simulink model "Fly_calculatedLm"  (R2017b)
settings: Solver=VariableStepAuto  StartTime=0.0  StopTime=1  MaxStep=1e-4  RelTol=1e-3
libraries: powerlib x17, powerlib_meascontrol x1
settings Model: Creator=yusuf  LastModifiedBy=SiF
settings CodeAppCC: StateflowObjectComments=on

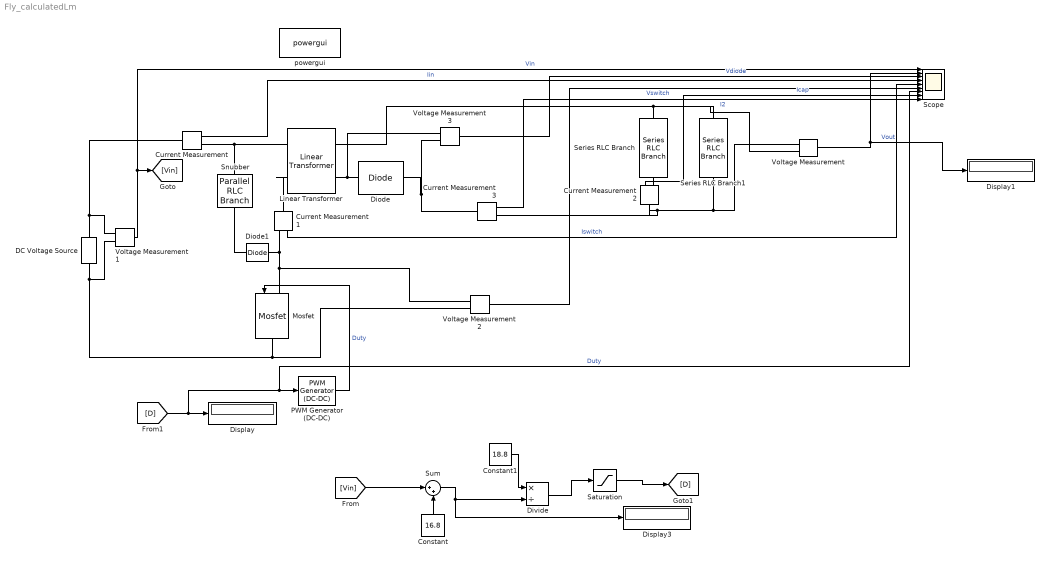
== system Fly_calculatedLm ==
  Constant : Constant  Value=16.8
  Constant1 : Constant  Value=18.8
  Current Measurement{,1..3} (4 alike) : powerlib/Measurements/Current Measurement  PhasorSimulation=off  OutputType=Complex  PSBequivalent=0
  DC Voltage Source : powerlib/Electrical Sources/DC Voltage Source  Amplitude=48  Measurements=None
  Diode : powerlib/Power Electronics/Diode  Ron=0.001  Lon=0  Vf=0.8  IC=0  UseSnubber=0  Rs=500  Cs=250e-9  Measurements=off
  Diode1 : powerlib/Power Electronics/Diode  Ron=0.001  Lon=0  Vf=0.8  IC=0  UseSnubber=0  Rs=500  Cs=250e-9  Measurements=off
  Display : Display
  Display1 : Display
  Display3 : Display
  Divide : Product  Inputs=*/
  Linear Transformer : powerlib/Elements/Linear Transformer  UNITS=SI  NominalPower=[100 32e3 ]  winding1=[60 0 12e-6]  winding2=[20 0 0]  ThreeWindings=off  winding3=[3.15e+05 0.7938 0.0001316]  RmLm=[1080.5 400e-6]  Measurements=Magnetization current  DataType=on
  Mosfet : powerlib/Power Electronics/Mosfet  Ron=0.1  Lon=0  Rd=0.01  Vfd=0  IC=0  Rs=1e5  Cs=inf  Measurements=off
  PWM Generator (DC-DC) : powerlib_meascontrol/Pulse & Signal Generators/PWM Generator (DC-DC)  Fsw=32000  Ts=0
  Saturation : Saturate  UpperLimit=0.85  LowerLimit=0
  Scope : Scope  NumInputPorts=9
  Series RLC Branch : powerlib/Elements/Series RLC Branch  LConnTagsString=__new0  RConnTagsString=__new0  BranchType=C  Resistance=1  Inductance=1e-3  SetiL0=off  InitialCurrent=0  Capacitance=1e-3  Setx0=off  InitialVoltage=0  Measurements=None
  Series RLC Branch1 : powerlib/Elements/Series RLC Branch  LConnTagsString=__new0  RConnTagsString=__new0  BranchType=R  Resistance=5/6  Inductance=1e-3  SetiL0=off  InitialCurrent=0  Capacitance=1e-6  Setx0=off  InitialVoltage=0  Measurements=None
  Snubber : powerlib/Elements/Parallel RLC Branch  LConnTagsString=a  RConnTagsString=__new0  BranchType=RC  Resistance=10e3  Inductance=1e-3  SetiL0=off  InitialCurrent=0  Capacitance=47e-9  Setx0=off  InitialVoltage=0  Measurements=None
  Sum : Sum  Inputs=|++
  Voltage Measurement{,1..3} (4 alike) : powerlib/Measurements/Voltage Measurement  PhasorSimulation=off  OutputType=Complex  PSBequivalent=0
  powergui : powerlib/powergui  Priority=1  SimulationMode=Continuous  SampleTime=50e-6  frequency=60  Iterations=50  frequencyindice=0  Pbase=100e6  ErrMax=1e-4  UnitsV=kV  UnitsW=MW  buscounter=0  FunctionMessages=off  echomessages=off  EnableUseOfTLC=off  CurrentSourceSwitches=off  DisableSnubberDevices=off  DisableRonSwitches=off  DisableVfSwitches=off  DisplayEquations=off  SolverType=Tustin/Backward Euler (TBE)  Interpol=off  ExternalGateDelay=off  methode=off  Ts=100  x0status=blocks  SPID=on  SwTol=0  HookPort=off  RestoreLinks=warning  ResistiveCurrentMeasurement=off  Frange=[0:2:500]  Ylog=off  Xlog=on  ShowGrid=off  save=off  variable=ZData  structure=0  ZoomFFT=off  StartTime=0.0  cycles=1  DisplayStyle=1  fundamental=60  FreqAxis=off  MaxFrequency=1000  frequencyindicesteady=1  RmsSteady=1  display=off
  wires:
  [D] -> Display/1, Scope/7, PWM Generator (DC-DC)/1  "Duty"
  PWM Generator (DC-DC)/1 -> Mosfet/1  "Duty"
  Voltage Measurement/1 -> Display1/1, Scope/2  "Vout"
  Current Measurement/1 -> Scope/4  "Iin"
  Voltage Measurement1/1 -> [Vin], Scope/1  "Vin"
  Current Measurement1/1 -> Scope/5  "Iswitch"
  Voltage Measurement2/1 -> Scope/6  "Vswitch"
  Current Measurement2/1 -> Scope/8  "Icap"
  [Vin] -> Sum/1
  Constant/1 -> Sum/2
  Sum/1 -> Divide/2, Display3/1
  Saturation/1 -> [D]
  Constant1/1 -> Divide/1
  Divide/1 -> Saturation/1
  Voltage Measurement3/1 -> Scope/3  "Vdiode"
  Current Measurement3/1 -> Scope/9  "I2"
  connections:
  Mosfet/RConn1 -- Voltage Measurement2/LConn2 -- Voltage Measurement1/LConn2 -- DC Voltage Source/LConn1
  Linear Transformer/RConn1 -- Voltage Measurement/LConn2 -- Series RLC Branch1/RConn1 -- Series RLC Branch/RConn1
  Diode/LConn1 -- Voltage Measurement3/LConn1 -- Linear Transformer/RConn2
  Current Measurement2/LConn1 -- Current Measurement3/RConn1 -- Series RLC Branch1/LConn1 -- Voltage Measurement/LConn1
  DC Voltage Source/RConn1 -- Voltage Measurement1/LConn1 -- Current Measurement/LConn1
  Current Measurement/RConn1 -- Snubber/LConn1 -- Linear Transformer/LConn1
  Linear Transformer/LConn2 -- Current Measurement1/LConn1
  Current Measurement2/RConn1 -- Series RLC Branch/LConn1
  Diode1/RConn1 -- Snubber/RConn1
  Voltage Measurement3/LConn2 -- Current Measurement3/LConn1 -- Diode/RConn1
  Mosfet/LConn1 -- Voltage Measurement2/LConn1 -- Diode1/LConn1 -- Current Measurement1/RConn1
